simulink model "fuelPuddle"  (Simulink 3.00)
settings: Solver=ode45  StartTime=0.0  StopTime=100  RelTol=1e-3
undefined symbols (not defined in the file or in its folder): tau, x
settings Model: ExternalInput=[t,u]  SaveState=on  SaveOutput=off  LastModifiedBy=rconnors

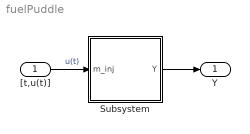
== system fuelPuddle ==
  "[t,u(t)]" : Inport  Port=1  PortWidth=-1  SampleTime=-1  DataType=auto
      settings: SignalType=auto
  Subsystem : Subsystem  mask{tau=tau, x=x}
      mask prompts: tau "Evaporation const"; x "Fuel Fraction"
  Y : Outport  Port=1
  wires:
  "[t,u(t)]"/1 -> Subsystem/1(m_inj)  "u(t)"
  Subsystem/1(Y) -> Y/1

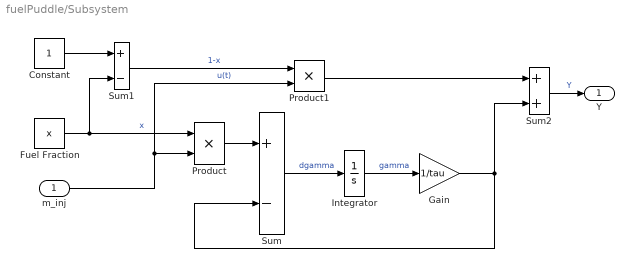
== system fuelPuddle/Subsystem ==
  m_inj : Inport  Port=1  PortWidth=-1  SampleTime=-1  DataType=auto
      settings: SignalType=auto
  Constant : Constant  Value=1
  Fuel Fraction : Constant  Value=x
  Gain : Gain  Gain=1/tau  SaturateOnIntegerOverflow=on
  Integrator : Integrator  ExternalReset=none  InitialConditionSource=internal  InitialCondition=0  LimitOutput=off  UpperSaturationLimit=inf  LowerSaturationLimit=-inf  ShowSaturationPort=off  ShowStatePort=off  AbsoluteTolerance=auto
  Product : Product  Inputs=2  SaturateOnIntegerOverflow=on
  Product1 : Product  Inputs=2  SaturateOnIntegerOverflow=on
  Sum : Sum  Inputs=+-  SaturateOnIntegerOverflow=on
  Sum1 : Sum  Inputs=+-  SaturateOnIntegerOverflow=on
  Sum2 : Sum  Inputs=++  SaturateOnIntegerOverflow=on
  Y : Outport  Port=1
  wires:
  Sum/1 -> Integrator/1  "dgamma"
  Product/1 -> Sum/1
  Constant/1 -> Sum1/1
  Fuel Fraction/1 -> Sum1/2, Product/1  "x"
  Sum1/1 -> Product1/1  "1-x"
  m_inj/1 -> Product/2, Product1/2  "u(t)"
  Product1/1 -> Sum2/1
  Sum2/1 -> Y/1  "Y"
  Integrator/1 -> Gain/1  "gamma"
  Gain/1 -> Sum/2, Sum2/2
